simulink model "full_maneuver_single_veh"  (R2020a)
settings: Solver=VariableStepAuto  StartTime=0.0  StopTime=90  FixedStep=0.1  MaxStep=5e-2  RelTol=1e-3
InitFcn:
  | totalVehicles = 5;
  | if exist('vehStatesBus', 'var')==0
  | load vehBuses
  | end
  | if exist('vehErrorsBus', 'var')==0
  | load vehBuses
  | end
libraries: simulink x69, powerlib_meascontrol x6, autolibshared x6, dspsigops x3, eeGeneralControl x2
(part 6 of 6)

== matlab function full_maneuver_single_veh/Fo/Regular Vehicle Following/switch/MATLAB Function ==
  data: h input; maxGap output; d0 input; vRef input; ev input; ehDot input; ea input; Kp parameter; Kd parameter; Ka parameter; Kdd parameter
function maxGap = followingGapThreshold(h, d0, vRef, ev, ehDot, ea, Kp, Kd, Ka, Kdd)

maxGap = h*vRef + d0 - 1/Kp*(Kd*ev + Kdd*ehDot + Ka*ea);

== matlab function full_maneuver_single_veh/Fo/findLeader/Subsystem/MATLAB Function ==
  data: ego input Bus: vehStatesBus; allVehicles input; leaderIdx output
function leaderIdx  = findLeader(ego, allVehicles)

nv = length(allVehicles);

leaderIdx = nv+1;

farAwayVehicle.X = ego.X + 10^4;
farAwayVehicle.Y = ego.Y;
farAwayVehicle.Xdot = ego.Xdot;
farAwayVehicle.u = 0;

leader = farAwayVehicle;
% For non lane changing vehicles, the leader is whoever is longitudinally
% closer and with any part of the body in the same lane.
% 1.8m (half lane) + 0.9m (half veh width)
for n = 1:nv
    if allVehicles(n).X>ego.X
        if abs(allVehicles(n).Y - ego.Y)<=2.7 && allVehicles(n).X<leader.X
            leaderIdx = n;
        end
    end
end

== matlab function full_maneuver_single_veh/Fd/Platoon Gap Generation Management/assignExtraSpace ==
  data: strategy input; extraSpaceFlag output; posInPlatoon input; platoonState input
function extraSpaceFlag = assignExtraSpace(strategy, posInPlatoon, platoonState)

myState = platoonState(posInPlatoon);

%%% Single vehicle case %%%
if length(platoonState)==1 
    extraSpaceFlag = myState<5;
    return
end

%%% Platoon case %%%
switch strategy
    case {1, 2}
        if posInPlatoon == 1
            followerState = platoonState(posInPlatoon+1);
            extraSpaceFlag = myState<5 || followerState<6; %any(platoonState<5)
        elseif posInPlatoon == length(platoonState)
            leaderState = platoonState(posInPlatoon-1);
            extraSpaceFlag = leaderState>1 && myState<5;
        else
            leaderState = platoonState(posInPlatoon-1);
            followerState = platoonState(posInPlatoon+1);
            extraSpaceFlag = leaderState>1 && (myState<5 || followerState<6);
        end
%     case 2
%         if posInPlatoon == 1
%             extraSpaceFlag = true;
%         else
%             extraSpaceFlag = platoonState(posInPlatoon-1)>5;
%         end
    case 3
        if posInPlatoon == length(platoonState)
            extraSpaceFlag = myState<5 || platoonState(1)<5;%any(platoonState<5)
            % eventually try platoonState(end-1)<5
        else
           followerState = platoonState(posInPlatoon+1); 
           extraSpaceFlag = followerState>4 && (myState<5 || followerState<6);
        end 
    otherwise
        error('Unknown strategy')
end

== matlab function full_maneuver_single_veh/Fd/Platoon Gap Generation Management/assignvirtualLeader ==
  data: strategy input; virtualLeaderFlag output; posInPlatoon input; platoonState input
function virtualLeaderFlag = assignVirtualLeader(strategy, posInPlatoon, platoonState)

myState = platoonState(posInPlatoon);

%%% Single vehicle case %%%
if length(platoonState)==1 
    virtualLeaderFlag = myState<5;
    return
end

%%% Platoon case %%%
switch strategy
    case {1, 2}
        if posInPlatoon == 1
            virtualLeaderFlag = myState<5;
        else
            leaderState = platoonState(posInPlatoon-1);
            virtualLeaderFlag = leaderState>3 && myState<5 ;
        end
    case 3
        if posInPlatoon == 1
           followerState = platoonState(posInPlatoon+1);
           virtualLeaderFlag = followerState>4 && (myState<5 || followerState<6);
        elseif posInPlatoon == length(platoonState)
            leaderState = platoonState(posInPlatoon-1);
            virtualLeaderFlag = myState<5 || leaderState<5;
            % first condition is redundant since leaderState won't change
            % if myState<5 - leaving it there for clarity and completeness
        else
           leaderState = platoonState(posInPlatoon-1); 
           followerState = platoonState(posInPlatoon+1);
           virtualLeaderFlag = followerState>4 && (myState<5 || leaderState<5);
        end 
    otherwise
        error('Unknown strategy')
end

== matlab function full_maneuver_single_veh/Fd/Regular Vehicle Following/switch free flow/MATLAB Function ==
  data: h input; maxGap output; d0 input; vRef input; ev input; ehDot input; ea input; Kp parameter; Kd parameter; Ka parameter; Kdd parameter
function maxGap = followingGapThreshold(h, d0, vRef, ev, ehDot, ea, Kp, Kd, Ka, Kdd)

maxGap = h*vRef + d0 - 1/Kp*(Kd*ev + Kdd*ehDot + Ka*ea);

== matlab function full_maneuver_single_veh/Fd/Virtual Follower Manager/determineVirtualFollower ==
  data: nVehicles input; posInPlatoon input; lcStrategy input; virtualFollowerIdx output
function virtualFollowerIdx  = ...
    determineVirtualFollower(nVehicles, posInPlatoon, lcStrategy)

% Important assumption:
% The array of vehicles is ordered as [Ld, Fd, Lo, p1, ..., pN, Fo]

% To consider: would it be more organized to have two vehicle arrays (one 
% for each lane)?

switch lcStrategy
    case {1, 2} % synchronous, leader changes first
        virtualFollowerIdx = 2;
    case 3 % last veh changes first
        if posInPlatoon == nVehicles-4
            virtualFollowerIdx = 2;
        else
            virtualFollowerIdx = 3 + (posInPlatoon + 1);
        end
    otherwise
        error('[determineVirtualFollower in Simulink model] Unknown lane changing strategy]')
end

end

== matlab function full_maneuver_single_veh/Fd/Virtual Leader Manager/determineVirtualLeader ==
  data: nVehicles input; lcFlag input; lcDone input; virtualLeaderIdx output; posInPlatoon input; lcStrategy input
function virtualLeaderIdx  = ...
    determineVirtualLeader(nVehicles, lcFlag, lcDone, posInPlatoon, lcStrategy)

% Important assumption:
% The array of vehicles is ordered as [Ld, Fd, Lo, p1, ..., pN, Fo]

% To consider: would it be more organized to have two vehicle arrays (one 
% for each lane)?

if ~lcFlag% gap generating vehicle
    virtualLeaderIdx = nVehicles-1; % last platoon vehicle
    
else % lane changing vehicle
    switch lcStrategy
        case {1, 2} % synchronous, leader changes first
            if posInPlatoon == 1
                virtualLeaderIdx = 1;
            else
                virtualLeaderIdx = 3 + (posInPlatoon - 1);
            end
            
        case 3 % last veh changes first
            if ~lcDone
                virtualLeaderIdx = 1;
            else
                if posInPlatoon == 1
                    virtualLeaderIdx = 1;
                else
                    virtualLeaderIdx = 3 + (posInPlatoon - 1);
                end
            end
            
        otherwise
            error('[determineVirtualLeader in Simulink model] Unknown lane changing strategy]')
    end
end

end

== matlab function full_maneuver_single_veh/Fd/Virtual Vehicle Following/switch min vel/MATLAB Function ==
  data: h input; maxGap output; d0 input; vRef input; ev input; ehDot input; ea input; Kp parameter; Kd parameter; Ka parameter; Kdd parameter
function maxGap = followingGapThreshold(h, d0, vRef, ev, ehDot, ea, Kp, Kd, Ka, Kdd)

maxGap = h*vRef + d0 - 1/Kp*(Kd*ev + Kdd*ehDot + Ka*ea);

== stateflow chart full_maneuver_single_veh/Fd_bkp/ControlChoice ==
  state RegVehFoll
    entry:
    state = 0;
    during:
    u = regFollInput;
  state AdjForLaneChange
    during:
    if ~xor(leaderInRange, vLeaderInRange)
    state = 1;
    u = min(regFollInput, virtualFollInput);
    elseif vLeaderInRange
    state = 2;
    u = virtualFollInput;
    else
    state = 3;
    u = regFollInput;
    end
  (default) -> RegVehFoll
  AdjForLaneChange -> RegVehFoll : [~vLeaderAssigned]
  RegVehFoll -> AdjForLaneChange : [startAdj && vLeaderAssigned]
  data: startAdj input; vLeaderAssigned input; regFollInput input; leaderInRange input; u output; virtualFollInput input; vLeaderInRange input; state output

== matlab function full_maneuver_single_veh/Fd_bkp/Find Leader/Subsystem/MATLAB Function ==
  data: ego input Bus: vehStatesBus; allVehicles input; leaderIdx output
function leaderIdx  = findLeader(ego, allVehicles)

nv = length(allVehicles);

leaderIdx = nv+1;

farAwayVehicle.X = ego.X + 10^4;
farAwayVehicle.Y = ego.Y;
farAwayVehicle.Xdot = ego.Xdot;
farAwayVehicle.u = 0;

leader = farAwayVehicle;
% For non lane changing vehicles, the leader is whoever is longitudinally
% closer and with any part of the body in the same lane.
% 1.8m (half lane) + 0.9m (half veh width)
for n = 1:nv
    if allVehicles(n).X>ego.X
        if abs(allVehicles(n).Y - ego.Y)<=2.7 && allVehicles(n).X<leader.X
            leaderIdx = n;
        end
    end
end

== matlab function full_maneuver_single_veh/Ld/Regular Vehicle Following/switch/MATLAB Function ==
  data: h input; maxGap output; d0 input; vRef input; ev input; ehDot input; ea input; Kp parameter; Kd parameter; Ka parameter; Kdd parameter
function maxGap = followingGapThreshold(h, d0, vRef, ev, ehDot, ea, Kp, Kd, Ka, Kdd)

maxGap = h*vRef + d0 - 1/Kp*(Kd*ev + Kdd*ehDot + Ka*ea);

== matlab function full_maneuver_single_veh/Fd_bkp/Platoon Gap Generation Management/assignExtraSpace ==
  data: strategy input; extraSpaceFlag output; posInPlatoon input; platoonState input
function extraSpaceFlag = assignExtraSpace(strategy, posInPlatoon, platoonState)

myState = platoonState(posInPlatoon);

%%% Single vehicle case %%%
if length(platoonState)==1 
    extraSpaceFlag = myState<5;
    return
end

%%% Platoon case %%%
switch strategy
    case {1, 2}
        if posInPlatoon == 1
            followerState = platoonState(posInPlatoon+1);
            extraSpaceFlag = myState<5 || followerState<6; %any(platoonState<5)
        elseif posInPlatoon == length(platoonState)
            leaderState = platoonState(posInPlatoon-1);
            extraSpaceFlag = leaderState>1 && myState<5;
        else
            leaderState = platoonState(posInPlatoon-1);
            followerState = platoonState(posInPlatoon+1);
            extraSpaceFlag = leaderState>1 && (myState<5 || followerState<6);
        end
%     case 2
%         if posInPlatoon == 1
%             extraSpaceFlag = true;
%         else
%             extraSpaceFlag = platoonState(posInPlatoon-1)>5;
%         end
    case 3
        if posInPlatoon == length(platoonState)
            extraSpaceFlag = myState<5 || platoonState(1)<5;%any(platoonState<5)
            % eventually try platoonState(end-1)<5
        else
           followerState = platoonState(posInPlatoon+1); 
           extraSpaceFlag = followerState>4 && (myState<5 || followerState<6);
        end 
    otherwise
        error('Unknown strategy')
end

== matlab function full_maneuver_single_veh/Fd_bkp/Platoon Gap Generation Management/assignvirtualLeader ==
  data: strategy input; virtualLeaderFlag output; posInPlatoon input; platoonState input
function virtualLeaderFlag = assignVirtualLeader(strategy, posInPlatoon, platoonState)

myState = platoonState(posInPlatoon);

%%% Single vehicle case %%%
if length(platoonState)==1 
    virtualLeaderFlag = myState<5;
    return
end

%%% Platoon case %%%
switch strategy
    case {1, 2}
        if posInPlatoon == 1
            virtualLeaderFlag = myState<5;
        else
            leaderState = platoonState(posInPlatoon-1);
            virtualLeaderFlag = leaderState>3 && myState<5 ;
        end
    case 3
        if posInPlatoon == 1
           followerState = platoonState(posInPlatoon+1);
           virtualLeaderFlag = followerState>4 && (myState<5 || followerState<6);
        elseif posInPlatoon == length(platoonState)
            leaderState = platoonState(posInPlatoon-1);
            virtualLeaderFlag = myState<5 || leaderState<5;
            % first condition is redundant since leaderState won't change
            % if myState<5 - leaving it there for clarity and completeness
        else
           leaderState = platoonState(posInPlatoon-1); 
           followerState = platoonState(posInPlatoon+1);
           virtualLeaderFlag = followerState>4 && (myState<5 || leaderState<5);
        end 
    otherwise
        error('Unknown strategy')
end
